simulink model "electricalModel"  (R2025a)
settings: Solver=VariableStepAuto  StartTime=0.0  StopTime=10.0  RelTol=1e-3
libraries: myBatteries_lib x64, fl_lib x2, nesl_utility x2
settings Model: Creator=mbhattu  LastModifiedBy=mbhattu

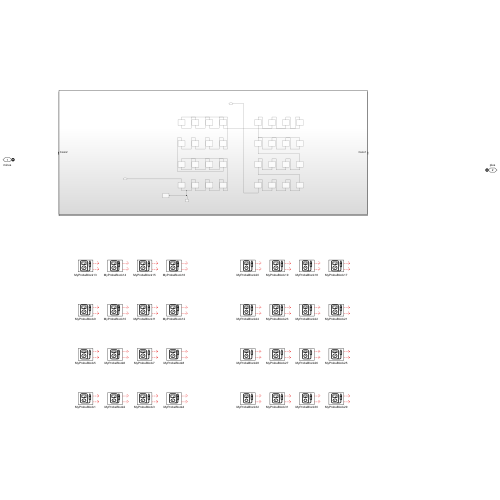
[thumbnail: Simulink's stored preview of the top-level diagram]
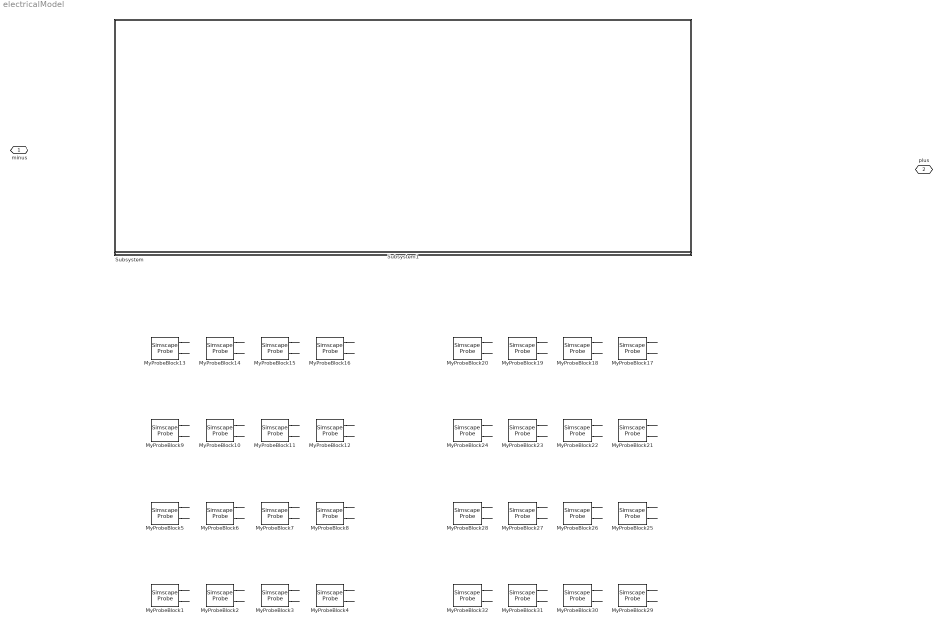
== system electricalModel ==
  MyProbeBlock1 : SimscapeProbe  BoundBlock=1  Variables="{\"Cell1.ocv\":{\"Probing\":\"ON\"},\"socCell\":{\"Probing\":\"ON\"}}"
  MyProbeBlock10 : SimscapeProbe  BoundBlock=10  Variables="{\"Cell1.ocv\":{\"Probing\":\"ON\"},\"socCell\":{\"Probing\":\"ON\"}}"
  MyProbeBlock11 : SimscapeProbe  BoundBlock=11  Variables="{\"Cell1.ocv\":{\"Probing\":\"ON\"},\"socCell\":{\"Probing\":\"ON\"}}"
  MyProbeBlock12 : SimscapeProbe  BoundBlock=12  Variables="{\"Cell1.ocv\":{\"Probing\":\"ON\"},\"socCell\":{\"Probing\":\"ON\"}}"
  MyProbeBlock13 : SimscapeProbe  BoundBlock=13  Variables="{\"Cell1.ocv\":{\"Probing\":\"ON\"},\"socCell\":{\"Probing\":\"ON\"}}"
  MyProbeBlock14 : SimscapeProbe  BoundBlock=14  Variables="{\"Cell1.ocv\":{\"Probing\":\"ON\"},\"socCell\":{\"Probing\":\"ON\"}}"
  MyProbeBlock15 : SimscapeProbe  BoundBlock=15  Variables="{\"Cell1.ocv\":{\"Probing\":\"ON\"},\"socCell\":{\"Probing\":\"ON\"}}"
  MyProbeBlock16 : SimscapeProbe  BoundBlock=16  Variables="{\"Cell1.ocv\":{\"Probing\":\"ON\"},\"socCell\":{\"Probing\":\"ON\"}}"
  MyProbeBlock17 : SimscapeProbe  BoundBlock=17  Variables="{\"Cell1.ocv\":{\"Probing\":\"ON\"},\"socCell\":{\"Probing\":\"ON\"}}"
  MyProbeBlock18 : SimscapeProbe  BoundBlock=18  Variables="{\"Cell1.ocv\":{\"Probing\":\"ON\"},\"socCell\":{\"Probing\":\"ON\"}}"
  MyProbeBlock19 : SimscapeProbe  BoundBlock=19  Variables="{\"Cell1.ocv\":{\"Probing\":\"ON\"},\"socCell\":{\"Probing\":\"ON\"}}"
  MyProbeBlock2 : SimscapeProbe  BoundBlock=2  Variables="{\"Cell1.ocv\":{\"Probing\":\"ON\"},\"socCell\":{\"Probing\":\"ON\"}}"
  MyProbeBlock20 : SimscapeProbe  BoundBlock=20  Variables="{\"Cell1.ocv\":{\"Probing\":\"ON\"},\"socCell\":{\"Probing\":\"ON\"}}"
  MyProbeBlock21 : SimscapeProbe  BoundBlock=21  Variables="{\"Cell1.ocv\":{\"Probing\":\"ON\"},\"socCell\":{\"Probing\":\"ON\"}}"
  MyProbeBlock22 : SimscapeProbe  BoundBlock=22  Variables="{\"Cell1.ocv\":{\"Probing\":\"ON\"},\"socCell\":{\"Probing\":\"ON\"}}"
  MyProbeBlock23 : SimscapeProbe  BoundBlock=23  Variables="{\"Cell1.ocv\":{\"Probing\":\"ON\"},\"socCell\":{\"Probing\":\"ON\"}}"
  MyProbeBlock24 : SimscapeProbe  BoundBlock=24  Variables="{\"Cell1.ocv\":{\"Probing\":\"ON\"},\"socCell\":{\"Probing\":\"ON\"}}"
  MyProbeBlock25 : SimscapeProbe  BoundBlock=25  Variables="{\"Cell1.ocv\":{\"Probing\":\"ON\"},\"socCell\":{\"Probing\":\"ON\"}}"
  MyProbeBlock26 : SimscapeProbe  BoundBlock=26  Variables="{\"Cell1.ocv\":{\"Probing\":\"ON\"},\"socCell\":{\"Probing\":\"ON\"}}"
  MyProbeBlock27 : SimscapeProbe  BoundBlock=27  Variables="{\"Cell1.ocv\":{\"Probing\":\"ON\"},\"socCell\":{\"Probing\":\"ON\"}}"
  MyProbeBlock28 : SimscapeProbe  BoundBlock=28  Variables="{\"Cell1.ocv\":{\"Probing\":\"ON\"},\"socCell\":{\"Probing\":\"ON\"}}"
  MyProbeBlock29 : SimscapeProbe  BoundBlock=29  Variables="{\"Cell1.ocv\":{\"Probing\":\"ON\"},\"socCell\":{\"Probing\":\"ON\"}}"
  MyProbeBlock3 : SimscapeProbe  BoundBlock=3  Variables="{\"Cell1.ocv\":{\"Probing\":\"ON\"},\"socCell\":{\"Probing\":\"ON\"}}"
  MyProbeBlock30 : SimscapeProbe  BoundBlock=30  Variables="{\"Cell1.ocv\":{\"Probing\":\"ON\"},\"socCell\":{\"Probing\":\"ON\"}}"
  MyProbeBlock31 : SimscapeProbe  BoundBlock=31  Variables="{\"Cell1.ocv\":{\"Probing\":\"ON\"},\"socCell\":{\"Probing\":\"ON\"}}"
  MyProbeBlock32 : SimscapeProbe  BoundBlock=32  Variables="{\"Cell1.ocv\":{\"Probing\":\"ON\"},\"socCell\":{\"Probing\":\"ON\"}}"
  MyProbeBlock4 : SimscapeProbe  BoundBlock=4  Variables="{\"Cell1.ocv\":{\"Probing\":\"ON\"},\"socCell\":{\"Probing\":\"ON\"}}"
  MyProbeBlock5 : SimscapeProbe  BoundBlock=5  Variables="{\"Cell1.ocv\":{\"Probing\":\"ON\"},\"socCell\":{\"Probing\":\"ON\"}}"
  MyProbeBlock6 : SimscapeProbe  BoundBlock=6  Variables="{\"Cell1.ocv\":{\"Probing\":\"ON\"},\"socCell\":{\"Probing\":\"ON\"}}"
  MyProbeBlock7 : SimscapeProbe  BoundBlock=7  Variables="{\"Cell1.ocv\":{\"Probing\":\"ON\"},\"socCell\":{\"Probing\":\"ON\"}}"
  MyProbeBlock8 : SimscapeProbe  BoundBlock=8  Variables="{\"Cell1.ocv\":{\"Probing\":\"ON\"},\"socCell\":{\"Probing\":\"ON\"}}"
  MyProbeBlock9 : SimscapeProbe  BoundBlock=9  Variables="{\"Cell1.ocv\":{\"Probing\":\"ON\"},\"socCell\":{\"Probing\":\"ON\"}}"
  Subsystem : Subsystem
  Subsystem1 : Subsystem
  minus : PMIOPort  Side=Left
  plus : PMIOPort  Port=2  Side=Left
  wires:
  MyProbeBlock25/2 -> ?
  MyProbeBlock29/2 -> ?
  MyProbeBlock3/1 -> ?
  MyProbeBlock12/2 -> ?
  MyProbeBlock1/2 -> ?
  MyProbeBlock11/2 -> ?
  MyProbeBlock1/1 -> ?
  MyProbeBlock11/1 -> ?
  MyProbeBlock27/2 -> ?
  MyProbeBlock28/2 -> ?
  MyProbeBlock29/1 -> ?
  MyProbeBlock23/2 -> ?
  MyProbeBlock23/1 -> ?
  MyProbeBlock30/1 -> ?
  MyProbeBlock22/2 -> ?
  MyProbeBlock10/2 -> ?
  MyProbeBlock4/2 -> ?
  MyProbeBlock3/2 -> ?
  MyProbeBlock5/2 -> ?
  MyProbeBlock12/1 -> ?
  MyProbeBlock6/1 -> ?
  MyProbeBlock22/1 -> ?
  MyProbeBlock18/1 -> ?
  MyProbeBlock25/1 -> ?
  MyProbeBlock28/1 -> ?
  MyProbeBlock32/2 -> ?
  MyProbeBlock19/2 -> ?
  MyProbeBlock24/1 -> ?
  MyProbeBlock15/2 -> ?
  MyProbeBlock14/2 -> ?
  MyProbeBlock8/1 -> ?
  MyProbeBlock21/1 -> ?
  MyProbeBlock16/2 -> ?
  MyProbeBlock26/2 -> ?
  MyProbeBlock4/1 -> ?
  MyProbeBlock9/1 -> ?
  MyProbeBlock13/1 -> ?
  MyProbeBlock27/1 -> ?
  MyProbeBlock20/2 -> ?
  MyProbeBlock7/1 -> ?
  MyProbeBlock16/1 -> ?
  MyProbeBlock8/2 -> ?
  MyProbeBlock17/1 -> ?
  MyProbeBlock32/1 -> ?
  MyProbeBlock17/2 -> ?
  MyProbeBlock31/1 -> ?
  MyProbeBlock20/1 -> ?
  MyProbeBlock13/2 -> ?
  MyProbeBlock15/1 -> ?
  MyProbeBlock2/1 -> ?
  MyProbeBlock7/2 -> ?
  MyProbeBlock24/2 -> ?
  MyProbeBlock26/1 -> ?
  MyProbeBlock5/1 -> ?
  MyProbeBlock21/2 -> ?
  MyProbeBlock31/2 -> ?
  MyProbeBlock18/2 -> ?
  MyProbeBlock6/2 -> ?
  MyProbeBlock9/2 -> ?
  MyProbeBlock14/1 -> ?
  MyProbeBlock2/2 -> ?
  MyProbeBlock30/2 -> ?
  MyProbeBlock19/1 -> ?
  MyProbeBlock10/1 -> ?

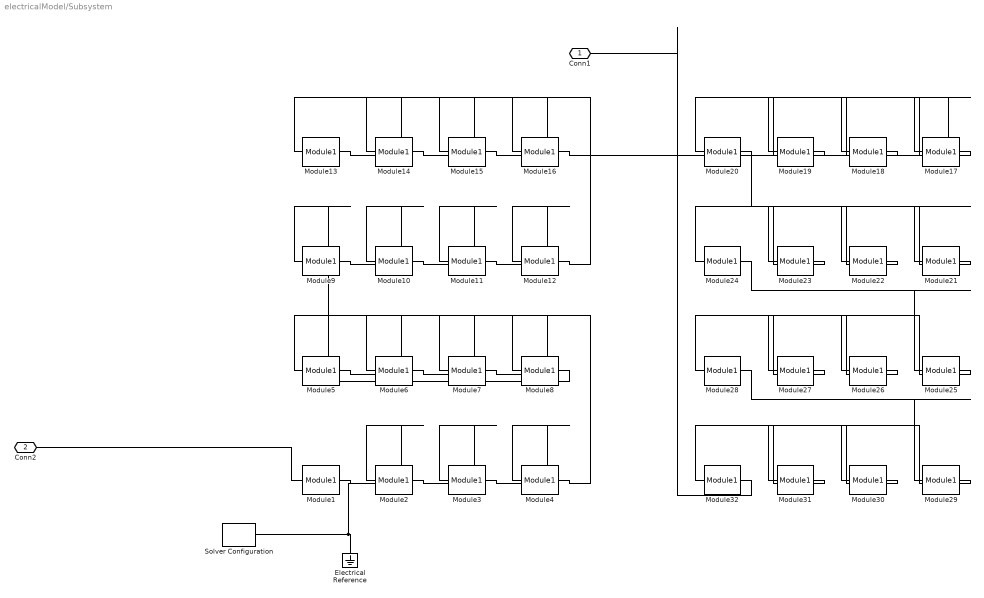
== system electricalModel/Subsystem ==
  Electrical Reference : fl_lib/Electrical/Electrical Elements/Electrical Reference
  Module{1..32} (32 alike) : myBatteries_lib/Module1  SOC_vecCell=[0, .1, .25, .5, .75, .9, 1]  V0_vecCell=[3.5057, 3.566, 3.6337, 3.7127, 3.9259, 4.0777, 4.1928] V  V_rangeCell=[0, inf] V  R0_vecCell=[.0085, .0085, .0087, .0082, .0083, .0085, .0085] Ohm  AHCell=27 A*hr  extrapolation_optionCell=simscape.enum.extrapolation.nearest  P=2  S=6  iCell_specify=off  iCell_priority=None  iCell=0 A  iCell_nominal_specify=off  iCell_nominal_value=1  iCell_nominal_unit=A  vCell_specify=off  vCell_priority=None  vCell=0 V  vCell_nominal_specify=off  vCell_nominal_value=1  vCell_nominal_unit=V  socCell_specify=off  socCell_priority=High  socCell=1  socCell_nominal_specify=off  socCell_nominal_value=1  socCell_nominal_unit=1  numCyclesCell_specify=off  numCyclesCell_priority=High  numCyclesCell=0  numCyclesCell_nominal_specify=off  numCyclesCell_nominal_value=1  numCyclesCell_nominal_unit=1  vParallelAssembly_specify=off  vParallelAssembly_priority=None  vParallelAssembly=repmat(0, 6, 1) V  vParallelAssembly_nominal_specify=off  vParallelAssembly_nominal_value=1  vParallelAssembly_nominal_unit=V  socParallelAssembly_specify=off  socParallelAssembly_priority=None  socParallelAssembly=repmat(1, 6, 1)  socParallelAssembly_nominal_specify=off  socParallelAssembly_nominal_value=1  socParallelAssembly_nominal_unit=1
      settings: InternalSimscapePortConfiguration="{\"Bottom\":[{\"id\":\"n\",\"label\":\"-\",\"type\":\"foundation.electrical.electrical\"}],\"Left\":[],\"Right\":[],\"Top\":[{\"id\":\"p\",\"label\":\"+\",\"type\":\"foundation.electrical.electrical\"}]}"
  Solver Configuration : nesl_utility/Solver Configuration  PhysicalDomain=network_engine_domain  SubClassName=solver  LeftPortType=input  RightPortType=generic  Tones=[]  Harmonics=[]  SimulateNoise=off  Profile=off  UseLocalSampling=off  EnableSwitchedLinearOptims=on  FrequencyDomain=off  UseCCode=off  RelTol=0.001  AbsTol=0.001  MinStep=1e-09  ToWorkspace=off  RevertToSquareIcSolve=off  NumHomotopyIterations=100  PhasorMode=off  PhasorModeNumHarmonics=1  ConsistencySolver=NEWTON_XTOL_AFTER_FTOL  IndexReductionMethod=DerivativeReplacement  DoDC=off  ResidualTolerance=1e-09  ConsistencyTolSource=GLOBAL  ConsistencyAbsTol=0.001  ConsistencyRelTol=0.001  ConsistencyTolFactor=0.001  UseLocalSolver=off  LocalSolverChoice=NE_BACKWARD_EULER_ADVANCER  ResolveIndetEquations=on  FunctionEvalNumThread=1  LocalSolverSampleTime=0.001  DoFixedCost=off  MaxNonlinIter=3  MaxModeIter=2  ComputeImpulses=off  ImpulseIterations=2  LinearAlgebra=auto  LinearAlgebraNumThread=0  EquationFormulation=NE_TIME_EF  DelaysMemoryBudget=1024  AutomaticFiltering=on  FilteringTimeConstant=0.001  PartitionStorageMethod=AS_NEEDED  PartitionMemoryBudget=1024  PartitionMethod=ROBUST  MultibodyUseLocalSolver=off  MultibodyLocalSolverChoice=ODE1  MultibodyLocalSolverSampleTime=0.001
  Conn1 : PMIOPort  Side=Right
  Conn2 : PMIOPort  Port=2  Side=Left
  connections:
  Module8/RConn1 -- Module9/LConn1
  Module3/RConn1 -- Module4/LConn1
  Module21/RConn1 -- Module22/LConn1
  Module11/RConn1 -- Module12/LConn1
  Module22/RConn1 -- Module23/LConn1
  Module14/RConn1 -- Module15/LConn1
  Module1/RConn1 -- Solver Configuration/RConn1 -- Electrical Reference/LConn1 -- Module2/LConn1
  Module28/RConn1 -- Module29/LConn1
  Module20/RConn1 -- Module21/LConn1
  Module25/RConn1 -- Module26/LConn1
  Module16/RConn1 -- Module17/LConn1
  Module31/RConn1 -- Module32/LConn1
  Module18/RConn1 -- Module19/LConn1
  Module15/RConn1 -- Module16/LConn1
  Module30/RConn1 -- Module31/LConn1
  Module10/RConn1 -- Module11/LConn1
  Module32/RConn1 -- Conn1/RConn1
  Module23/RConn1 -- Module24/LConn1
  Module6/RConn1 -- Module7/LConn1
  Module29/RConn1 -- Module30/LConn1
  Module24/RConn1 -- Module25/LConn1
  Module12/RConn1 -- Module13/LConn1
  Module9/RConn1 -- Module10/LConn1
  Module5/RConn1 -- Module6/LConn1
  Module4/RConn1 -- Module5/LConn1
  Module19/RConn1 -- Module20/LConn1
  Module27/RConn1 -- Module28/LConn1
  Module17/RConn1 -- Module18/LConn1
  Module13/RConn1 -- Module14/LConn1
  Module26/RConn1 -- Module27/LConn1
  Module7/RConn1 -- Module8/LConn1
  Module2/RConn1 -- Module3/LConn1
  Module1/LConn1 -- Conn2/RConn1

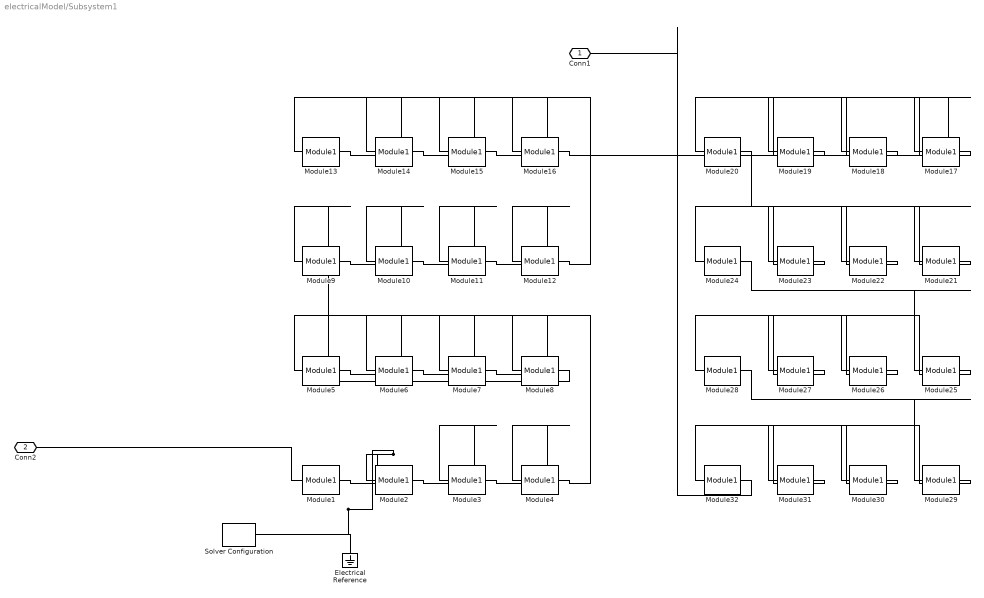
== system electricalModel/Subsystem1 ==
  Electrical Reference : fl_lib/Electrical/Electrical Elements/Electrical Reference
  Module{1..32} (32 alike) : myBatteries_lib/Module1  SOC_vecCell=[0, .1, .25, .5, .75, .9, 1]  V0_vecCell=[3.5057, 3.566, 3.6337, 3.7127, 3.9259, 4.0777, 4.1928] V  V_rangeCell=[0, inf] V  R0_vecCell=[.0085, .0085, .0087, .0082, .0083, .0085, .0085] Ohm  AHCell=27 A*hr  extrapolation_optionCell=simscape.enum.extrapolation.nearest  P=2  S=6  iCell_specify=off  iCell_priority=None  iCell=0 A  iCell_nominal_specify=off  iCell_nominal_value=1  iCell_nominal_unit=A  vCell_specify=off  vCell_priority=None  vCell=0 V  vCell_nominal_specify=off  vCell_nominal_value=1  vCell_nominal_unit=V  socCell_specify=off  socCell_priority=High  socCell=1  socCell_nominal_specify=off  socCell_nominal_value=1  socCell_nominal_unit=1  numCyclesCell_specify=off  numCyclesCell_priority=High  numCyclesCell=0  numCyclesCell_nominal_specify=off  numCyclesCell_nominal_value=1  numCyclesCell_nominal_unit=1  vParallelAssembly_specify=off  vParallelAssembly_priority=None  vParallelAssembly=repmat(0, 6, 1) V  vParallelAssembly_nominal_specify=off  vParallelAssembly_nominal_value=1  vParallelAssembly_nominal_unit=V  socParallelAssembly_specify=off  socParallelAssembly_priority=None  socParallelAssembly=repmat(1, 6, 1)  socParallelAssembly_nominal_specify=off  socParallelAssembly_nominal_value=1  socParallelAssembly_nominal_unit=1
      settings: InternalSimscapePortConfiguration="{\"Bottom\":[{\"id\":\"n\",\"label\":\"-\",\"type\":\"foundation.electrical.electrical\"}],\"Left\":[],\"Right\":[],\"Top\":[{\"id\":\"p\",\"label\":\"+\",\"type\":\"foundation.electrical.electrical\"}]}"
  Solver Configuration : nesl_utility/Solver Configuration  PhysicalDomain=network_engine_domain  SubClassName=solver  LeftPortType=input  RightPortType=generic  Tones=[]  Harmonics=[]  SimulateNoise=off  Profile=off  UseLocalSampling=off  EnableSwitchedLinearOptims=on  FrequencyDomain=off  UseCCode=off  RelTol=0.001  AbsTol=0.001  MinStep=1e-09  ToWorkspace=off  RevertToSquareIcSolve=off  NumHomotopyIterations=100  PhasorMode=off  PhasorModeNumHarmonics=1  ConsistencySolver=NEWTON_XTOL_AFTER_FTOL  IndexReductionMethod=DerivativeReplacement  DoDC=off  ResidualTolerance=1e-09  ConsistencyTolSource=GLOBAL  ConsistencyAbsTol=0.001  ConsistencyRelTol=0.001  ConsistencyTolFactor=0.001  UseLocalSolver=off  LocalSolverChoice=NE_BACKWARD_EULER_ADVANCER  ResolveIndetEquations=on  FunctionEvalNumThread=1  LocalSolverSampleTime=0.001  DoFixedCost=off  MaxNonlinIter=3  MaxModeIter=2  ComputeImpulses=off  ImpulseIterations=2  LinearAlgebra=auto  LinearAlgebraNumThread=0  EquationFormulation=NE_TIME_EF  DelaysMemoryBudget=1024  AutomaticFiltering=on  FilteringTimeConstant=0.001  PartitionStorageMethod=AS_NEEDED  PartitionMemoryBudget=1024  PartitionMethod=ROBUST  MultibodyUseLocalSolver=off  MultibodyLocalSolverChoice=ODE1  MultibodyLocalSolverSampleTime=0.001
  Conn1 : PMIOPort  Side=Right
  Conn2 : PMIOPort  Port=2  Side=Left
  connections:
  Module1/LConn1 -- Conn2/RConn1
  Module2/RConn1 -- Module3/LConn1
  Module7/RConn1 -- Module8/LConn1
  Module26/RConn1 -- Module27/LConn1
  Module13/RConn1 -- Module14/LConn1
  Module17/RConn1 -- Module18/LConn1
  Module27/RConn1 -- Module28/LConn1
  Module19/RConn1 -- Module20/LConn1
  Module4/RConn1 -- Module5/LConn1
  Module5/RConn1 -- Module6/LConn1
  Module9/RConn1 -- Module10/LConn1
  Module12/RConn1 -- Module13/LConn1
  Module24/RConn1 -- Module25/LConn1
  Module29/RConn1 -- Module30/LConn1
  Module6/RConn1 -- Module7/LConn1
  Module23/RConn1 -- Module24/LConn1
  Module32/RConn1 -- Conn1/RConn1
  Module10/RConn1 -- Module11/LConn1
  Module30/RConn1 -- Module31/LConn1
  Module15/RConn1 -- Module16/LConn1
  Module18/RConn1 -- Module19/LConn1
  Module31/RConn1 -- Module32/LConn1
  Module16/RConn1 -- Module17/LConn1
  Module25/RConn1 -- Module26/LConn1
  Module20/RConn1 -- Module21/LConn1
  Module28/RConn1 -- Module29/LConn1
  Module2/LConn1 -- Electrical Reference/LConn1 -- Solver Configuration/RConn1 -- Module1/RConn1
  Module14/RConn1 -- Module15/LConn1
  Module22/RConn1 -- Module23/LConn1
  Module11/RConn1 -- Module12/LConn1
  Module21/RConn1 -- Module22/LConn1
  Module3/RConn1 -- Module4/LConn1
  Module8/RConn1 -- Module9/LConn1
